simulink model "NInvState"  (R2024b)
settings: configuration reference "STM32H7_Config" (kept outside this file)
settings Model: DataDictionary=Master_Dictionary.sldd  EnableAccessToBaseWorkspace=off  Creator=torni  LastModifiedBy=William
settings ConfigSetRef: SourceName=STM32H7_Config

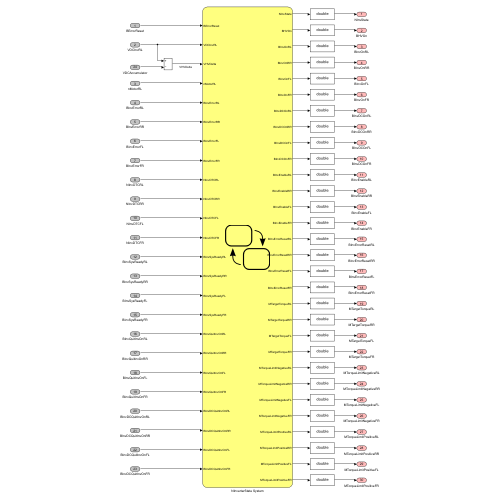
[thumbnail: Simulink's stored preview of the top-level diagram]
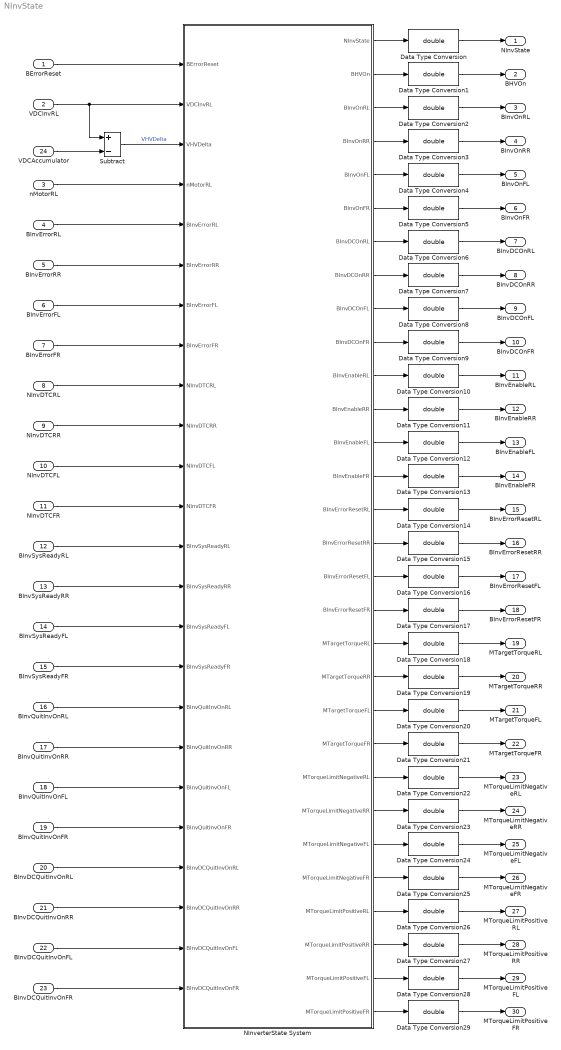
== system NInvState ==
  BErrorReset : Inport  OutDataTypeStr=boolean
  VDCInvRL : Inport  Port=2  OutDataTypeStr=double
  nMotorRL : Inport  Port=3  OutDataTypeStr=double
  BInvErrorRL : Inport  Port=4  OutDataTypeStr=boolean
  BInvErrorRR : Inport  Port=5  OutDataTypeStr=boolean
  BInvErrorFL : Inport  Port=6  OutDataTypeStr=boolean
  BInvErrorFR : Inport  Port=7  OutDataTypeStr=boolean
  NInvDTCRL : Inport  Port=8  OutDataTypeStr=double
  "NInvDTCRR " : Inport  Port=9  OutDataTypeStr=double
  NInvDTCFL : Inport  Port=10  OutDataTypeStr=double
  NInvDTCFR : Inport  Port=11  OutDataTypeStr=double
  BInvSysReadyRL : Inport  Port=12  OutDataTypeStr=boolean
  BInvSysReadyRR : Inport  Port=13  OutDataTypeStr=boolean
  BInvSysReadyFL : Inport  Port=14  OutDataTypeStr=boolean
  BInvSysReadyFR : Inport  Port=15  OutDataTypeStr=boolean
  BInvQuitInvOnRL : Inport  Port=16  OutDataTypeStr=boolean
  BInvQuitInvOnRR : Inport  Port=17  OutDataTypeStr=boolean
  BInvQuitInvOnFL : Inport  Port=18  OutDataTypeStr=boolean
  BInvQuitInvOnFR : Inport  Port=19  OutDataTypeStr=boolean
  BInvDCQuitInvOnRL : Inport  Port=20  OutDataTypeStr=boolean
  BInvDCQuitInvOnRR : Inport  Port=21  OutDataTypeStr=boolean
  BInvDCQuitInvOnFL : Inport  Port=22  OutDataTypeStr=boolean
  BInvDCQuitInvOnFR : Inport  Port=23  OutDataTypeStr=boolean
  VDCAccumulator : Inport  Port=24  OutDataTypeStr=double
  Data Type Conversion{,1..29} (30 alike) : DataTypeConversion  OutDataTypeStr=double  SaturateOnIntegerOverflow=off  RndMeth=Floor
  NInverterState System : Stateflow chart  TreatAsAtomicUnit=on
  Subtract : Sum  Inputs=+-
  NInvState : Outport  OutDataTypeStr=double  VectorParamsAs1DForOutWhenUnconnected=off
  BHVOn : Outport  Port=2  OutDataTypeStr=double  VectorParamsAs1DForOutWhenUnconnected=off
  BInvOnRL : Outport  Port=3  OutDataTypeStr=double  VectorParamsAs1DForOutWhenUnconnected=off
  BInvOnRR : Outport  Port=4  OutDataTypeStr=double  VectorParamsAs1DForOutWhenUnconnected=off
  BInvOnFL : Outport  Port=5  OutDataTypeStr=double  VectorParamsAs1DForOutWhenUnconnected=off
  BInvOnFR : Outport  Port=6  OutDataTypeStr=double  VectorParamsAs1DForOutWhenUnconnected=off
  BInvDCOnRL : Outport  Port=7  OutDataTypeStr=double  VectorParamsAs1DForOutWhenUnconnected=off
  BInvDCOnRR : Outport  Port=8  OutDataTypeStr=double  VectorParamsAs1DForOutWhenUnconnected=off
  BInvDCOnFL : Outport  Port=9  OutDataTypeStr=double  VectorParamsAs1DForOutWhenUnconnected=off
  BInvDCOnFR : Outport  Port=10  OutDataTypeStr=double  VectorParamsAs1DForOutWhenUnconnected=off
  BInvEnableRL : Outport  Port=11  OutDataTypeStr=double  VectorParamsAs1DForOutWhenUnconnected=off
  BInvEnableRR : Outport  Port=12  OutDataTypeStr=double  VectorParamsAs1DForOutWhenUnconnected=off
  BInvEnableFL : Outport  Port=13  OutDataTypeStr=double  VectorParamsAs1DForOutWhenUnconnected=off
  BInvEnableFR : Outport  Port=14  OutDataTypeStr=double  VectorParamsAs1DForOutWhenUnconnected=off
  BInvErrorResetRL : Outport  Port=15  OutDataTypeStr=double  VectorParamsAs1DForOutWhenUnconnected=off
  BInvErrorResetRR : Outport  Port=16  OutDataTypeStr=double  VectorParamsAs1DForOutWhenUnconnected=off
  BInvErrorResetFL : Outport  Port=17  OutDataTypeStr=double  VectorParamsAs1DForOutWhenUnconnected=off
  BInvErrorResetFR : Outport  Port=18  OutDataTypeStr=double  VectorParamsAs1DForOutWhenUnconnected=off
  MTargetTorqueRL : Outport  Port=19  OutDataTypeStr=double  VectorParamsAs1DForOutWhenUnconnected=off
  MTargetTorqueRR : Outport  Port=20  OutDataTypeStr=double  VectorParamsAs1DForOutWhenUnconnected=off
  MTargetTorqueFL : Outport  Port=21  OutDataTypeStr=double  VectorParamsAs1DForOutWhenUnconnected=off
  MTargetTorqueFR : Outport  Port=22  OutDataTypeStr=double  VectorParamsAs1DForOutWhenUnconnected=off
  MTorqueLimitNegativeRL : Outport  Port=23  OutDataTypeStr=double  VectorParamsAs1DForOutWhenUnconnected=off
  MTorqueLimitNegativeRR : Outport  Port=24  OutDataTypeStr=double  VectorParamsAs1DForOutWhenUnconnected=off
  MTorqueLimitNegativeFL : Outport  Port=25  OutDataTypeStr=double  VectorParamsAs1DForOutWhenUnconnected=off
  MTorqueLimitNegativeFR : Outport  Port=26  OutDataTypeStr=double  VectorParamsAs1DForOutWhenUnconnected=off
  MTorqueLimitPositiveRL : Outport  Port=27  OutDataTypeStr=double  VectorParamsAs1DForOutWhenUnconnected=off
  MTorqueLimitPositiveRR : Outport  Port=28  OutDataTypeStr=double  VectorParamsAs1DForOutWhenUnconnected=off
  MTorqueLimitPositiveFL : Outport  Port=29  OutDataTypeStr=double  VectorParamsAs1DForOutWhenUnconnected=off
  MTorqueLimitPositiveFR : Outport  Port=30  OutDataTypeStr=double  VectorParamsAs1DForOutWhenUnconnected=off
  wires:
  NInverterState System/2(BHVOn) -> Data Type Conversion1/1
  NInverterState System/1(NInvState) -> Data Type Conversion/1
  BErrorReset/1 -> NInverterState System/1(BErrorReset)
  VDCInvRL/1 -> NInverterState System/2(VDCInvRL), Subtract/1
  nMotorRL/1 -> NInverterState System/4(nMotorRL)
  BInvErrorRL/1 -> NInverterState System/5(BInvErrorRL)
  BInvErrorRR/1 -> NInverterState System/6(BInvErrorRR)
  BInvErrorFL/1 -> NInverterState System/7(BInvErrorFL)
  BInvErrorFR/1 -> NInverterState System/8(BInvErrorFR)
  NInvDTCRL/1 -> NInverterState System/9(NInvDTCRL)
  "NInvDTCRR "/1 -> NInverterState System/10(NInvDTCRR)
  NInvDTCFL/1 -> NInverterState System/11(NInvDTCFL)
  NInvDTCFR/1 -> NInverterState System/12(NInvDTCFR)
  BInvSysReadyRL/1 -> NInverterState System/13(BInvSysReadyRL)
  BInvSysReadyRR/1 -> NInverterState System/14(BInvSysReadyRR)
  BInvSysReadyFL/1 -> NInverterState System/15(BInvSysReadyFL)
  BInvSysReadyFR/1 -> NInverterState System/16(BInvSysReadyFR)
  BInvQuitInvOnRL/1 -> NInverterState System/17(BInvQuitInvOnRL)
  BInvQuitInvOnRR/1 -> NInverterState System/18(BInvQuitInvOnRR)
  BInvQuitInvOnFL/1 -> NInverterState System/19(BInvQuitInvOnFL)
  BInvQuitInvOnFR/1 -> NInverterState System/20(BInvQuitInvOnFR)
  BInvDCQuitInvOnRL/1 -> NInverterState System/21(BInvDCQuitInvOnRL)
  BInvDCQuitInvOnFL/1 -> NInverterState System/23(BInvDCQuitInvOnFL)
  BInvDCQuitInvOnRR/1 -> NInverterState System/22(BInvDCQuitInvOnRR)
  BInvDCQuitInvOnFR/1 -> NInverterState System/24(BInvDCQuitInvOnFR)
  VDCAccumulator/1 -> Subtract/2
  Subtract/1 -> NInverterState System/3(VHVDelta)  "VHVDelta"
  NInverterState System/19(MTargetTorqueRL) -> Data Type Conversion18/1
  NInverterState System/20(MTargetTorqueRR) -> Data Type Conversion19/1
  NInverterState System/21(MTargetTorqueFL) -> Data Type Conversion20/1
  NInverterState System/22(MTargetTorqueFR) -> Data Type Conversion21/1
  NInverterState System/23(MTorqueLimitNegativeRL) -> Data Type Conversion22/1
  NInverterState System/24(MTorqueLimitNegativeRR) -> Data Type Conversion23/1
  NInverterState System/25(MTorqueLimitNegativeFL) -> Data Type Conversion24/1
  NInverterState System/26(MTorqueLimitNegativeFR) -> Data Type Conversion25/1
  NInverterState System/27(MTorqueLimitPositiveRL) -> Data Type Conversion26/1
  NInverterState System/28(MTorqueLimitPositiveRR) -> Data Type Conversion27/1
  NInverterState System/29(MTorqueLimitPositiveFL) -> Data Type Conversion28/1
  NInverterState System/30(MTorqueLimitPositiveFR) -> Data Type Conversion29/1
  NInverterState System/18(BInvErrorResetFR) -> Data Type Conversion17/1
  NInverterState System/17(BInvErrorResetFL) -> Data Type Conversion16/1
  NInverterState System/16(BInvErrorResetRR) -> Data Type Conversion15/1
  NInverterState System/15(BInvErrorResetRL) -> Data Type Conversion14/1
  NInverterState System/14(BInvEnableFR) -> Data Type Conversion13/1
  NInverterState System/13(BInvEnableFL) -> Data Type Conversion12/1
  NInverterState System/12(BInvEnableRR) -> Data Type Conversion11/1
  NInverterState System/11(BInvEnableRL) -> Data Type Conversion10/1
  NInverterState System/10(BInvDCOnFR) -> Data Type Conversion9/1
  NInverterState System/9(BInvDCOnFL) -> Data Type Conversion8/1
  NInverterState System/8(BInvDCOnRR) -> Data Type Conversion7/1
  NInverterState System/7(BInvDCOnRL) -> Data Type Conversion6/1
  NInverterState System/6(BInvOnFR) -> Data Type Conversion5/1
  NInverterState System/5(BInvOnFL) -> Data Type Conversion4/1
  NInverterState System/4(BInvOnRR) -> Data Type Conversion3/1
  NInverterState System/3(BInvOnRL) -> Data Type Conversion2/1
  Data Type Conversion1/1 -> BHVOn/1
  Data Type Conversion/1 -> NInvState/1
  Data Type Conversion2/1 -> BInvOnRL/1
  Data Type Conversion3/1 -> BInvOnRR/1
  Data Type Conversion4/1 -> BInvOnFL/1
  Data Type Conversion5/1 -> BInvOnFR/1
  Data Type Conversion6/1 -> BInvDCOnRL/1
  Data Type Conversion7/1 -> BInvDCOnRR/1
  Data Type Conversion8/1 -> BInvDCOnFL/1
  Data Type Conversion9/1 -> BInvDCOnFR/1
  Data Type Conversion10/1 -> BInvEnableRL/1
  Data Type Conversion11/1 -> BInvEnableRR/1
  Data Type Conversion12/1 -> BInvEnableFL/1
  Data Type Conversion13/1 -> BInvEnableFR/1
  Data Type Conversion14/1 -> BInvErrorResetRL/1
  Data Type Conversion15/1 -> BInvErrorResetRR/1
  Data Type Conversion16/1 -> BInvErrorResetFL/1
  Data Type Conversion17/1 -> BInvErrorResetFR/1
  Data Type Conversion18/1 -> MTargetTorqueRL/1
  Data Type Conversion19/1 -> MTargetTorqueRR/1
  Data Type Conversion20/1 -> MTargetTorqueFL/1
  Data Type Conversion21/1 -> MTargetTorqueFR/1
  Data Type Conversion22/1 -> MTorqueLimitNegativeRL/1
  Data Type Conversion23/1 -> MTorqueLimitNegativeRR/1
  Data Type Conversion24/1 -> MTorqueLimitNegativeFL/1
  Data Type Conversion25/1 -> MTorqueLimitNegativeFR/1
  Data Type Conversion26/1 -> MTorqueLimitPositiveRL/1
  Data Type Conversion27/1 -> MTorqueLimitPositiveRR/1
  Data Type Conversion28/1 -> MTorqueLimitPositiveFL/1
  Data Type Conversion29/1 -> MTorqueLimitPositiveFR/1

== stateflow chart NInvState/NInverterState System ==
  state Inv_State_Idle
    entry:
    NInvState=0;
  state Inv_Error_Checks
    state Inv_LV_Check2
      entry:
      NInvState=2
      BInvErrorResetRR=0;
      BInvErrorResetRL=0;
      BInvErrorResetFR=0;
      BInvErrorResetFL=0;
    state Inv_LV_Check1
      entry:
      BInvErrorResetRR=1;
      BInvErrorResetRL=1;
      BInvErrorResetFR=1;
      BInvErrorResetFL=1;
    state Inv_LV_OK
      entry:
      NInvState=3;
    state Inv_LV_Check
      entry:
      NInvState=1;
      BInvErrorResetRR=0;
      BInvErrorResetRL=0;
      BInvErrorResetFR=0;
      BInvErrorResetFL=0;
    Inv_LV_Check1 -> Inv_LV_Check2 : after(100, tick)
        | [BInvErrorFL==0&&...
        | BInvErrorFR==0&&...
        | BInvErrorRR==0&&...
        | BInvErrorRL==0]
    (default) -> Inv_LV_Check
    Inv_LV_Check2 -> Inv_LV_Check [order 1] : [BInvErrorRR==1 &&...
        | BInvErrorRL==1 &&...
        | BInvErrorFR==1 &&...
        | BInvErrorFL==1]
    Inv_LV_Check2 -> Inv_LV_OK [order 2] : [BInvErrorRR==0 &&...
        | BInvErrorRL==0 &&...
        | BInvErrorFR==0 &&...
        | BInvErrorFL==0 &&...
        | BInvSysReadyRL==1 &&...
        | BInvSysReadyRR==1 &&...
        | BInvSysReadyFL==1 &&...
        | BInvSysReadyFR==1]
    Inv_LV_Check -> Inv_LV_Check1 : after(100,tick)
    Inv_LV_OK -> Inv_LV_Check : [BErrorReset==1 && nMotorRL<500]
  state Inv_OK
    entry:
    NInvState=92
  state Encoder_Reset_RL
    state Encoder_Error_RL
      entry:
      NInvState=404
      state PBX_SENSORS_ini
        entry:
        BInvErrorResetRL=0;
      state Error_On
        entry:
        BInvErrorResetRL=1;
      state Error_off
        entry:
        BInvErrorResetRL=0;
      (default) -> Encoder_Reset_RL.Encoder_Error_RL.PBX_SENSORS_ini
      Encoder_Reset_RL.Encoder_Error_RL.PBX_SENSORS_ini -> Encoder_Reset_RL.Encoder_Error_RL.Error_On : after(50, tick)
      Encoder_Reset_RL.Encoder_Error_RL.Error_off -> Encoder_Reset_RL.Encoder_Error_RL.PBX_SENSORS_ini [order 2] : [BInvErrorRL ==1]
      Encoder_Reset_RL.Encoder_Error_RL.Error_On -> Encoder_Reset_RL.Encoder_Error_RL.Error_off : after(100, tick)
          | [BInvErrorRL ==0]
    state Inverter_HV_Checks3
      exit:
      BHVOn=1
      state Inverter_IN
        entry:
        NInvState = 22
        BInvDCOnRL = 1
      state Inv_Error_Check_2
        BInvErrorResetRL = 0
        NInvState = 00
      state Inv_Error_Reset
        entry:
        NInvState = 00
        BInvErrorResetRL=1
        BInvDCOnRL=0
        BInvEnableRL = 0
        BInvOnRL = 0
      state START_UP
        entry:
        NInvState = 23
        MTargetTorqueRL=0
        MTorqueLimitNegativeRL = 0
        MTorqueLimitPositiveRL = 0
        BInvOnRL = 1
      state Inv_Error_Check_1
        entry:
        NInvState = 00
        MTorqueLimitNegativeRL = 0
        MTorqueLimitPositiveRL = 0
      state Inverter_ON
        entry:
        NInvState = 24
        BInvEnableRL = 1
      state TorqueReq_Ready
        entry:
        NInvState = 25
        MTorqueLimitNegativeRL = -100
        MTorqueLimitPositiveRL = 204.8
      (default) -> Encoder_Reset_RL.Inverter_HV_Checks3.Inverter_IN
      (junction 784) -> Encoder_Reset_RL.Inverter_HV_Checks3.Inverter_IN [order 1] : [BInvErrorRL==0]
      Encoder_Reset_RL.Inverter_HV_Checks3.Inv_Error_Check_2 -> (junction 784) : after(500,tick)
      (junction 784) -> Encoder_Reset_RL.Inverter_HV_Checks3.Inv_Error_Check_1 [order 2] : [BInvErrorRL==1]
      Encoder_Reset_RL.Inverter_HV_Checks3.Inv_Error_Reset -> Encoder_Reset_RL.Inverter_HV_Checks3.Inv_Error_Check_2 : after(500,tick)
      Encoder_Reset_RL.Inverter_HV_Checks3.Inverter_IN -> Encoder_Reset_RL.Inverter_HV_Checks3.START_UP : [BInvDCQuitInvOnRL==1]
      Encoder_Reset_RL.Inverter_HV_Checks3.START_UP -> Encoder_Reset_RL.Inverter_HV_Checks3.Inverter_ON : after(100,tick)
      Encoder_Reset_RL.Inverter_HV_Checks3.Inv_Error_Check_1 -> Encoder_Reset_RL.Inverter_HV_Checks3.Inv_Error_Reset : after(500,tick)
      Encoder_Reset_RL.Inverter_HV_Checks3.Inverter_ON -> Encoder_Reset_RL.Inverter_HV_Checks3.TorqueReq_Ready [order 1] : [BInvQuitInvOnRL == 1]
      Encoder_Reset_RL.Inverter_HV_Checks3.Inverter_ON -> Encoder_Reset_RL.Inverter_HV_Checks3.Inv_Error_Check_1 [order 2] : [BInvErrorRL==1]
      Encoder_Reset_RL.Inverter_HV_Checks3.TorqueReq_Ready -> Encoder_Reset_RL.Inverter_HV_Checks3.Inv_Error_Check_1 [order 1] : [BInvErrorRL==1]
    state Encoder_OK
      entry:
      NInvState = 26
    (default) -> Encoder_Error_RL
    Encoder_Reset_RL.Encoder_Error_RL.Error_off -> Encoder_Reset_RL.Inverter_HV_Checks3 [order 1] : [BInvSysReadyRL==1]
    Encoder_Reset_RL.Inverter_HV_Checks3.TorqueReq_Ready -> Encoder_Reset_RL.Encoder_OK [order 2] : [BInvErrorRL==0]
  state Encoder_Reset_RR
    state Encoder_Error_RR
      entry:
      NInvState = 404
      state PBX_SENSORS_ini
        entry:
        BInvErrorResetRR=0;
      state Error_On
        entry:
        BInvErrorResetRR=1;
      state Error_off
        entry:
        BInvErrorResetRR=0;
      (default) -> Encoder_Reset_RR.Encoder_Error_RR.PBX_SENSORS_ini
      Encoder_Reset_RR.Encoder_Error_RR.PBX_SENSORS_ini -> Encoder_Reset_RR.Encoder_Error_RR.Error_On : after(50, tick)
      Encoder_Reset_RR.Encoder_Error_RR.Error_off -> Encoder_Reset_RR.Encoder_Error_RR.PBX_SENSORS_ini [order 2] : [BInvErrorRR ==1]
      Encoder_Reset_RR.Encoder_Error_RR.Error_On -> Encoder_Reset_RR.Encoder_Error_RR.Error_off : after(100, tick)
          | [BInvErrorRR ==0]
    state Inverter_HV_CheckRR
      exit:
      BHVOn=1
      state Inverter_IN
        entry:
        NInvState = 27
        BInvDCOnRR = 1
      state Inv_Error_Check_2
        BInvErrorResetRR = 0
        NInvState = 00
      state Inv_Error_Reset
        entry:
        NInvState = 00
        BInvErrorResetRR=1
        BInvDCOnRR=0
        BInvEnableRR = 0
        BInvOnRR = 0
      state START_UP
        entry:
        NInvState = 28
        MTargetTorqueRR=0
        MTorqueLimitNegativeRR = 0
        MTorqueLimitPositiveRR = 0
        BInvOnRR = 1
      state Inv_Error_Check_1
        entry:
        NInvState = 00
        MTorqueLimitNegativeRR = 0
        MTorqueLimitPositiveRR = 0
      state Inverter_ON
        entry:
        NInvState = 29
        BInvEnableRR = 1
      state TorqueReq_Ready
        entry:
        NInvState = 30
        MTorqueLimitNegativeRR = -100
        MTorqueLimitPositiveRR = 204.8
      (default) -> Encoder_Reset_RR.Inverter_HV_CheckRR.Inverter_IN
      (junction 861) -> Encoder_Reset_RR.Inverter_HV_CheckRR.Inverter_IN [order 1] : [BInvErrorRR==0]
      Encoder_Reset_RR.Inverter_HV_CheckRR.Inv_Error_Check_2 -> (junction 861) : after(500,tick)
      (junction 861) -> Encoder_Reset_RR.Inverter_HV_CheckRR.Inv_Error_Check_1 [order 2] : [BInvErrorRR==1]
      Encoder_Reset_RR.Inverter_HV_CheckRR.Inv_Error_Reset -> Encoder_Reset_RR.Inverter_HV_CheckRR.Inv_Error_Check_2 : after(500,tick)
      Encoder_Reset_RR.Inverter_HV_CheckRR.Inverter_IN -> Encoder_Reset_RR.Inverter_HV_CheckRR.START_UP : [BInvDCQuitInvOnRR==1]
      Encoder_Reset_RR.Inverter_HV_CheckRR.START_UP -> Encoder_Reset_RR.Inverter_HV_CheckRR.Inverter_ON : after(100,tick)
      Encoder_Reset_RR.Inverter_HV_CheckRR.Inv_Error_Check_1 -> Encoder_Reset_RR.Inverter_HV_CheckRR.Inv_Error_Reset : after(500,tick)
      Encoder_Reset_RR.Inverter_HV_CheckRR.Inverter_ON -> Encoder_Reset_RR.Inverter_HV_CheckRR.TorqueReq_Ready [order 1] : [BInvQuitInvOnRR == 1]
      Encoder_Reset_RR.Inverter_HV_CheckRR.Inverter_ON -> Encoder_Reset_RR.Inverter_HV_CheckRR.Inv_Error_Check_1 [order 2] : [BInvErrorRR==1]
      Encoder_Reset_RR.Inverter_HV_CheckRR.TorqueReq_Ready -> Encoder_Reset_RR.Inverter_HV_CheckRR.Inv_Error_Check_1 [order 1] : [BInvErrorRR==1]
    state Encoder_OK
      entry:
      NInvState = 31
    (default) -> Encoder_Error_RR
    Encoder_Reset_RR.Encoder_Error_RR.Error_off -> Encoder_Reset_RR.Inverter_HV_CheckRR [order 1] : [BInvSysReadyRR==1]
    Encoder_Reset_RR.Inverter_HV_CheckRR.TorqueReq_Ready -> Encoder_Reset_RR.Encoder_OK [order 2] : [BInvErrorRR==0]
  state Encoder_Reset_FL
    state Encoder_Error_FL
      entry:
      NInvState = 404
      state Error_On
        entry:
        BInvErrorResetFL=1;
      state PBX_SENSORS_ini
        entry:
        BInvErrorResetFL=0;
      state Error_off
        entry:
        BInvErrorResetFL=0;
      (default) -> Encoder_Reset_FL.Encoder_Error_FL.PBX_SENSORS_ini
      Encoder_Reset_FL.Encoder_Error_FL.PBX_SENSORS_ini -> Encoder_Reset_FL.Encoder_Error_FL.Error_On : after(50, tick)
      Encoder_Reset_FL.Encoder_Error_FL.Error_off -> Encoder_Reset_FL.Encoder_Error_FL.PBX_SENSORS_ini [order 2] : [BInvErrorFL ==1]
      Encoder_Reset_FL.Encoder_Error_FL.Error_On -> Encoder_Reset_FL.Encoder_Error_FL.Error_off : after(100, tick)
          | [BInvErrorFL ==0]
    state Inverter_HV_Checks2
      exit:
      BHVOn=1
      state Inverter_IN
        entry:
        NInvState = 32
        BInvDCOnFL = 1
      state Inv_Error_Check_2
        BInvErrorResetFL = 0
        NInvState = 00
      state Inv_Error_Reset
        entry:
        NInvState = 00
        BInvErrorResetFL=1
        BInvDCOnFL=0
        BInvEnableFL = 0
        BInvOnFL = 0
      state START_UP
        entry:
        NInvState = 33
        MTargetTorqueFL=0
        MTorqueLimitNegativeFL = 0
        MTorqueLimitPositiveFL = 0
        BInvOnFL = 1
      state Inv_Error_Check_1
        entry:
        NInvState = 00
        MTorqueLimitNegativeFL = 0
        MTorqueLimitPositiveFL = 0
      state Inverter_ON
        entry:
        NInvState = 34
        BInvEnableFL = 1
      state TorqueReq_Ready
        entry:
        NInvState = 35
        MTorqueLimitNegativeFL = -100
        MTorqueLimitPositiveFL = 204.8
      (default) -> Encoder_Reset_FL.Inverter_HV_Checks2.Inverter_IN
      (junction 751) -> Encoder_Reset_FL.Inverter_HV_Checks2.Inverter_IN [order 1] : [BInvErrorFL==0]
      Encoder_Reset_FL.Inverter_HV_Checks2.Inv_Error_Check_2 -> (junction 751) : after(500,tick)
      (junction 751) -> Encoder_Reset_FL.Inverter_HV_Checks2.Inv_Error_Check_1 [order 2] : [BInvErrorFL==1]
      Encoder_Reset_FL.Inverter_HV_Checks2.Inv_Error_Reset -> Encoder_Reset_FL.Inverter_HV_Checks2.Inv_Error_Check_2 : after(500,tick)
      Encoder_Reset_FL.Inverter_HV_Checks2.Inverter_IN -> Encoder_Reset_FL.Inverter_HV_Checks2.START_UP : [BInvDCQuitInvOnFL==1]
      Encoder_Reset_FL.Inverter_HV_Checks2.START_UP -> Encoder_Reset_FL.Inverter_HV_Checks2.Inverter_ON : after(100,tick)
      Encoder_Reset_FL.Inverter_HV_Checks2.Inv_Error_Check_1 -> Encoder_Reset_FL.Inverter_HV_Checks2.Inv_Error_Reset : after(500,tick)
      Encoder_Reset_FL.Inverter_HV_Checks2.Inverter_ON -> Encoder_Reset_FL.Inverter_HV_Checks2.TorqueReq_Ready [order 1] : [BInvQuitInvOnFL == 1]
      Encoder_Reset_FL.Inverter_HV_Checks2.Inverter_ON -> Encoder_Reset_FL.Inverter_HV_Checks2.Inv_Error_Check_1 [order 2] : [BInvErrorFL==1]
      Encoder_Reset_FL.Inverter_HV_Checks2.TorqueReq_Ready -> Encoder_Reset_FL.Inverter_HV_Checks2.Inv_Error_Check_1 [order 1] : [BInvErrorFL==1]
    state Encoder_OK
      entry:
      NInvState = 36
    (default) -> Encoder_Error_FL
    Encoder_Reset_FL.Encoder_Error_FL.Error_off -> Inverter_HV_Checks2 [order 1] : [BInvSysReadyFL==1]
    Encoder_Reset_FL.Inverter_HV_Checks2.TorqueReq_Ready -> Encoder_Reset_FL.Encoder_OK [order 2] : [BInvErrorFL==0]
  state Inverter_HV_Checks
    state Inverter_HV_CheckFR
      exit:
      BHVOn=1;
      NInvState = 4
      state Inverter_IN
        entry:
        NInvState = 5
        BInvDCOnFR = 1
      state Inv_Error_Check_2
        BInvErrorResetFR = 0
        NInvState = 00;
      state Inv_Error_Reset
        entry:
        NInvState = 00
        BInvErrorResetFR=1
        BInvDCOnFR=0
        BInvEnableFR = 0
        BInvOnFR = 0
      state START_UP
        entry:
        NInvState = 6
        MTargetTorqueFR=0
        MTorqueLimitNegativeFR = 0
        MTorqueLimitPositiveFR = 0
        BInvOnFR = 1
      state Inv_Error_Check_1
        entry:
        NInvState = 00
        MTorqueLimitNegativeFR = 0
        MTorqueLimitPositiveFR = 0
      state Inverter_ON
        entry:
        NInvState = 7
        BInvEnableFR = 1
      state TorqueReq_Ready
        entry:
        NInvState = 8
        MTorqueLimitNegativeFR = -100
        MTorqueLimitPositiveFR = 204.8
      (default) -> Inverter_HV_Checks.Inverter_HV_CheckFR.Inverter_IN
      (junction 1179) -> Inverter_HV_Checks.Inverter_HV_CheckFR.Inverter_IN [order 1] : [BInvErrorFR==0]
      Inverter_HV_Checks.Inverter_HV_CheckFR.Inv_Error_Check_2 -> (junction 1179) : after(500,tick)
      (junction 1179) -> Inverter_HV_Checks.Inverter_HV_CheckFR.Inv_Error_Check_1 [order 2] : [BInvErrorFR==1]
      Inverter_HV_Checks.Inverter_HV_CheckFR.Inv_Error_Reset -> Inverter_HV_Checks.Inverter_HV_CheckFR.Inv_Error_Check_2 : after(500,tick)
      Inverter_HV_Checks.Inverter_HV_CheckFR.Inverter_IN -> Inverter_HV_Checks.Inverter_HV_CheckFR.START_UP : [BInvDCQuitInvOnFR==1]
      Inverter_HV_Checks.Inverter_HV_CheckFR.START_UP -> Inverter_HV_Checks.Inverter_HV_CheckFR.Inverter_ON : after(100,tick)
      Inverter_HV_Checks.Inverter_HV_CheckFR.Inv_Error_Check_1 -> Inverter_HV_Checks.Inverter_HV_CheckFR.Inv_Error_Reset : after(500,tick)
      Inverter_HV_Checks.Inverter_HV_CheckFR.Inverter_ON -> Inverter_HV_Checks.Inverter_HV_CheckFR.TorqueReq_Ready [order 1] : [BInvQuitInvOnFR == 1]
      Inverter_HV_Checks.Inverter_HV_CheckFR.Inverter_ON -> Inverter_HV_Checks.Inverter_HV_CheckFR.Inv_Error_Check_1 [order 2] : [BInvErrorFR==1]
      Inverter_HV_Checks.Inverter_HV_CheckFR.TorqueReq_Ready -> Inverter_HV_Checks.Inverter_HV_CheckFR.Inv_Error_Check_1 [order 2] : [BInvErrorFR==1]
    state Inv_HV_Check
    note: FRONT RIGHT INVERTER
    state Inverter_HV_CheckRR
      exit:
      BHVOn=1
      state Inverter_IN
        entry:
        NInvState = 9;
        BInvDCOnRR = 1
      state Inv_Error_Check_2
        BInvErrorResetRR = 0
      state Inv_Error_Reset
        entry:
        BInvErrorResetRR=1
        BInvDCOnRR=0
        BInvEnableRR = 0
        BInvOnRR = 0
      state START_UP
        entry:
        NInvState = 10
        MTargetTorqueRR=0
        MTorqueLimitNegativeRR = 0
        MTorqueLimitPositiveRR = 0
        BInvOnRR = 1
      state Inv_Error_Check_1
        entry:
        MTorqueLimitNegativeRR = 0
        MTorqueLimitPositiveRR = 0
      state Inverter_ON
        entry:
        NInvState = 11
        BInvEnableRR = 1
      state TorqueReq_Ready
        entry:
        NInvState = 12
        MTorqueLimitNegativeRR = -100
        MTorqueLimitPositiveRR = 204.8
      (default) -> Inverter_HV_Checks.Inverter_HV_CheckRR.Inverter_IN
      (junction 1201) -> Inverter_HV_Checks.Inverter_HV_CheckRR.Inverter_IN [order 1] : [BInvErrorRR==0]
      Inverter_HV_Checks.Inverter_HV_CheckRR.Inv_Error_Check_2 -> (junction 1201) : after(500,tick)
      (junction 1201) -> Inverter_HV_Checks.Inverter_HV_CheckRR.Inv_Error_Check_1 [order 2] : [BInvErrorRR==1]
      Inverter_HV_Checks.Inverter_HV_CheckRR.Inv_Error_Reset -> Inverter_HV_Checks.Inverter_HV_CheckRR.Inv_Error_Check_2 : after(500,tick)
      Inverter_HV_Checks.Inverter_HV_CheckRR.Inverter_IN -> Inverter_HV_Checks.Inverter_HV_CheckRR.START_UP : [BInvDCQuitInvOnRR==1]
      Inverter_HV_Checks.Inverter_HV_CheckRR.START_UP -> Inverter_HV_Checks.Inverter_HV_CheckRR.Inverter_ON : after(100,tick)
      Inverter_HV_Checks.Inverter_HV_CheckRR.Inv_Error_Check_1 -> Inverter_HV_Checks.Inverter_HV_CheckRR.Inv_Error_Reset : after(500,tick)
      Inverter_HV_Checks.Inverter_HV_CheckRR.Inverter_ON -> Inverter_HV_Checks.Inverter_HV_CheckRR.TorqueReq_Ready [order 1] : [BInvQuitInvOnRR == 1]
      Inverter_HV_Checks.Inverter_HV_CheckRR.Inverter_ON -> Inverter_HV_Checks.Inverter_HV_CheckRR.Inv_Error_Check_1 [order 2] : [BInvErrorRR==1]
      Inverter_HV_Checks.Inverter_HV_CheckRR.TorqueReq_Ready -> Inverter_HV_Checks.Inverter_HV_CheckRR.Inv_Error_Check_1 [order 2] : [BInvErrorRR==1]
    note: REAR RIGHT INVERTER
    state Inverter_HV_ChecksFL
      exit:
      BHVOn=1
      state Inverter_IN
        entry:
        NInvState = 13
        BInvDCOnFL = 1
      state Inv_Error_Check_2
        BInvErrorResetFL = 0
      state Inv_Error_Reset
        entry:
        BInvErrorResetFL=1
        BInvDCOnFL=0
        BInvEnableFL = 0
        BInvOnFL = 0
      state START_UP
        entry:
        NInvState = 14
        MTargetTorqueFL=0
        MTorqueLimitNegativeFL = 0
        MTorqueLimitPositiveFL = 0
        BInvOnFL = 1
      state Inv_Error_Check_1
        entry:
        MTorqueLimitNegativeFL = 0
        MTorqueLimitPositiveFL = 0
      state Inverter_ON
        entry:
        NInvState = 15
        BInvEnableFL = 1
      state TorqueReq_Ready
        entry:
        NInvState = 16
        MTorqueLimitNegativeFL = -100
        MTorqueLimitPositiveFL = 204.8
      (default) -> Inverter_HV_Checks.Inverter_HV_ChecksFL.Inverter_IN
      (junction 1222) -> Inverter_HV_Checks.Inverter_HV_ChecksFL.Inverter_IN [order 1] : [BInvErrorFL==0]
      Inverter_HV_Checks.Inverter_HV_ChecksFL.Inv_Error_Check_2 -> (junction 1222) : after(500,tick)
      (junction 1222) -> Inverter_HV_Checks.Inverter_HV_ChecksFL.Inv_Error_Check_1 [order 2] : [BInvErrorFL==1]
      Inverter_HV_Checks.Inverter_HV_ChecksFL.Inv_Error_Reset -> Inverter_HV_Checks.Inverter_HV_ChecksFL.Inv_Error_Check_2 : after(500,tick)
      Inverter_HV_Checks.Inverter_HV_ChecksFL.Inverter_IN -> Inverter_HV_Checks.Inverter_HV_ChecksFL.START_UP : [BInvDCQuitInvOnFL==1]
      Inverter_HV_Checks.Inverter_HV_ChecksFL.START_UP -> Inverter_HV_Checks.Inverter_HV_ChecksFL.Inverter_ON : after(100,tick)
      Inverter_HV_Checks.Inverter_HV_ChecksFL.Inv_Error_Check_1 -> Inverter_HV_Checks.Inverter_HV_ChecksFL.Inv_Error_Reset : after(500,tick)
      Inverter_HV_Checks.Inverter_HV_ChecksFL.Inverter_ON -> Inverter_HV_Checks.Inverter_HV_ChecksFL.TorqueReq_Ready [order 1] : [BInvQuitInvOnFL == 1]
      Inverter_HV_Checks.Inverter_HV_ChecksFL.Inverter_ON -> Inverter_HV_Checks.Inverter_HV_ChecksFL.Inv_Error_Check_1 [order 2] : [BInvErrorFL==1]
      Inverter_HV_Checks.Inverter_HV_ChecksFL.TorqueReq_Ready -> Inverter_HV_Checks.Inverter_HV_ChecksFL.Inv_Error_Check_1 [order 2] : [BInvErrorFL==1]
    note: FRONT LEFT INVERTER
    state Inverter_HV_ChecksRL
      exit:
      BHVOn=1
      state Inverter_IN
        entry:
        NInvState = 17
        BInvDCOnRL = 1
      state Inv_Error_Check_2
        BInvErrorResetRL = 0
      state Inv_Error_Reset
        entry:
        BInvErrorResetRL=1
        BInvDCOnRL=0
        BInvEnableRL = 0
        BInvOnRL = 0
      state START_UP
        entry:
        NInvState = 18
        MTargetTorqueRL=0
        MTorqueLimitNegativeRL = 0
        MTorqueLimitPositiveRL = 0
        BInvOnRL = 1
      state Inv_Error_Check_1
        entry:
        MTorqueLimitNegativeRL = 0
        MTorqueLimitPositiveRL = 0
      state Inverter_ON
        entry:
        NInvState = 19
        BInvEnableRL = 1
      state TorqueReq_Ready
        entry:
        NInvState = 20
        MTorqueLimitNegativeRL = -100
        MTorqueLimitPositiveRL = 204.8
      (default) -> Inverter_HV_Checks.Inverter_HV_ChecksRL.Inverter_IN
      (junction 1243) -> Inverter_HV_Checks.Inverter_HV_ChecksRL.Inverter_IN [order 1] : [BInvErrorRL==0]
      Inverter_HV_Checks.Inverter_HV_ChecksRL.Inv_Error_Check_2 -> (junction 1243) : after(500,tick)
      (junction 1243) -> Inverter_HV_Checks.Inverter_HV_ChecksRL.Inv_Error_Check_1 [order 2] : [BInvErrorRL==1]
      Inverter_HV_Checks.Inverter_HV_ChecksRL.Inv_Error_Reset -> Inverter_HV_Checks.Inverter_HV_ChecksRL.Inv_Error_Check_2 : after(500,tick)
      Inverter_HV_Checks.Inverter_HV_ChecksRL.Inverter_IN -> Inverter_HV_Checks.Inverter_HV_ChecksRL.START_UP : [BInvDCQuitInvOnRL==1]
      Inverter_HV_Checks.Inverter_HV_ChecksRL.START_UP -> Inverter_HV_Checks.Inverter_HV_ChecksRL.Inverter_ON : after(100,tick)
      Inverter_HV_Checks.Inverter_HV_ChecksRL.Inv_Error_Check_1 -> Inverter_HV_Checks.Inverter_HV_ChecksRL.Inv_Error_Reset : after(500,tick)
      Inverter_HV_Checks.Inverter_HV_ChecksRL.Inverter_ON -> Inverter_HV_Checks.Inverter_HV_ChecksRL.TorqueReq_Ready [order 1] : [BInvQuitInvOnRL == 1]
      Inverter_HV_Checks.Inverter_HV_ChecksRL.Inverter_ON -> Inverter_HV_Checks.Inverter_HV_ChecksRL.Inv_Error_Check_1 [order 2] : [BInvErrorRL==1]
      Inverter_HV_Checks.Inverter_HV_ChecksRL.TorqueReq_Ready -> Inverter_HV_Checks.Inverter_HV_ChecksRL.Inv_Error_Check_1 [order 1] : [BInvErrorRL==1]
    note: REAR LEFT INVERTER
    state Inv_OK
      entry:
      NInvState = 21;
    (default) -> Inv_HV_Check
    Inv_HV_Check -> Inverter_HV_CheckFR : [NInvState==3]
    Inverter_HV_Checks.Inverter_HV_CheckFR.TorqueReq_Ready -> Inverter_HV_Checks.Inverter_HV_CheckRR [order 1] : after(500,tick)[BInvErrorFR==0]
    Inverter_HV_Checks.Inverter_HV_CheckRR.TorqueReq_Ready -> Inverter_HV_ChecksFL [order 1] : after(500,tick)[BInvErrorRR==0]
    Inverter_HV_Checks.Inverter_HV_ChecksFL.TorqueReq_Ready -> Inverter_HV_ChecksRL [order 1] : after(500,tick)[BInvErrorFL==0]
    Inverter_HV_Checks.Inverter_HV_ChecksRL.TorqueReq_Ready -> Inverter_HV_Checks.Inv_OK [order 2] : [BInvErrorRL==0]
  state Encoder_Reset_FR
    state Encoder_Error_FR
      entry:
      NInvState = 404
      state PBX_SENSORS_ini
        entry:
        BInvErrorResetFR=0;
      state Error_On
        entry:
        BInvErrorResetFR=1;
      state Error_off
        entry:
        BInvErrorResetFR=0;
      (default) -> Encoder_Reset_FR.Encoder_Error_FR.PBX_SENSORS_ini
      Encoder_Reset_FR.Encoder_Error_FR.PBX_SENSORS_ini -> Encoder_Reset_FR.Encoder_Error_FR.Error_On : after(50, tick)
      Encoder_Reset_FR.Encoder_Error_FR.Error_off -> Encoder_Reset_FR.Encoder_Error_FR.PBX_SENSORS_ini [order 2] : [BInvErrorFR ==1]
      Encoder_Reset_FR.Encoder_Error_FR.Error_On -> Encoder_Reset_FR.Encoder_Error_FR.Error_off : after(100, tick)
          | [BInvErrorFR ==0]
    state Inverter_HV_Checks3
      exit:
      BHVOn=1
      state Inverter_IN
        entry:
        NInvState = 37
        BInvDCOnFR = 1
      state Inv_Error_Check_2
        BInvErrorResetFR = 0
        NInvState = 00
      state Inv_Error_Reset
        entry:
        NInvState = 00
        BInvErrorResetFR=1
        BInvDCOnFR=0
        BInvEnableFR = 0
        BInvOnFR = 0
      state START_UP
        entry:
        NInvState = 38
        MTargetTorqueFR=0
        MTorqueLimitNegativeFR = 0
        MTorqueLimitPositiveFR = 0
        BInvOnFR = 1
      state Inv_Error_Check_1
        entry:
        NInvState = 00
        MTorqueLimitNegativeFR = 0
        MTorqueLimitPositiveFR = 0
      state Inverter_ON
        entry:
        NInvState = 39
        BInvEnableFR = 1
      state TorqueReq_Ready
        entry:
        NInvState = 40
        MTorqueLimitNegativeFR = -100
        MTorqueLimitPositiveFR = 204.8
      (default) -> Encoder_Reset_FR.Inverter_HV_Checks3.Inverter_IN
      (junction 718) -> Encoder_Reset_FR.Inverter_HV_Checks3.Inverter_IN [order 1] : [BInvErrorFR==0]
      Encoder_Reset_FR.Inverter_HV_Checks3.Inv_Error_Check_2 -> (junction 718) : after(500,tick)
      (junction 718) -> Encoder_Reset_FR.Inverter_HV_Checks3.Inv_Error_Check_1 [order 2] : [BInvErrorFR==1]
      Encoder_Reset_FR.Inverter_HV_Checks3.Inv_Error_Reset -> Encoder_Reset_FR.Inverter_HV_Checks3.Inv_Error_Check_2 : after(500,tick)
      Encoder_Reset_FR.Inverter_HV_Checks3.Inverter_IN -> Encoder_Reset_FR.Inverter_HV_Checks3.START_UP : [BInvDCQuitInvOnFR==1]
      Encoder_Reset_FR.Inverter_HV_Checks3.START_UP -> Encoder_Reset_FR.Inverter_HV_Checks3.Inverter_ON : after(100,tick)
      Encoder_Reset_FR.Inverter_HV_Checks3.Inv_Error_Check_1 -> Encoder_Reset_FR.Inverter_HV_Checks3.Inv_Error_Reset : after(500,tick)
      Encoder_Reset_FR.Inverter_HV_Checks3.Inverter_ON -> Encoder_Reset_FR.Inverter_HV_Checks3.TorqueReq_Ready [order 1] : [BInvQuitInvOnFR == 1]
      Encoder_Reset_FR.Inverter_HV_Checks3.Inverter_ON -> Encoder_Reset_FR.Inverter_HV_Checks3.Inv_Error_Check_1 [order 2] : [BInvErrorFR==1]
      Encoder_Reset_FR.Inverter_HV_Checks3.TorqueReq_Ready -> Encoder_Reset_FR.Inverter_HV_Checks3.Inv_Error_Check_1 [order 1] : [BInvErrorFR==1]
    state Encoder_OK
      entry:
      NInvState = 41
    (default) -> Encoder_Error_FR
    Encoder_Reset_FR.Encoder_Error_FR.Error_off -> Encoder_Reset_FR.Inverter_HV_Checks3 [order 1] : [BInvSysReadyFR==1]
    Encoder_Reset_FR.Inverter_HV_Checks3.TorqueReq_Ready -> Encoder_Reset_FR.Encoder_OK [order 2] : [BInvErrorFR==0]
  (default) -> Inv_State_Idle
  Inv_State_Idle -> Inv_Error_Checks : [after (7000,tick)]
  Inv_OK -> Inv_State_Idle [order 6] : [VDCInvRL<60]
  Inv_OK -> Inv_Error_Checks [order 1] : [BErrorReset==1]
  Encoder_Reset_RL -> Inv_OK : [NInvState == 26]
  Inv_OK -> Encoder_Reset_RL [order 3] : [NInvDTCRL~=0 &&...
      | NInvDTCRL~=1049]
  Inverter_HV_Checks -> Inv_Error_Checks [order 1] : [BErrorReset==1]
  Inv_Error_Checks -> Inverter_HV_Checks : [VDCInvRL>60&&...
      | abs(VHVDelta)<10]
  Encoder_Reset_RR -> Inv_OK : [NInvState == 31]
  Inv_OK -> Encoder_Reset_RR [order 5] : [NInvDTCRR~=0 &&...
      | NInvDTCRR~=1049]
  Encoder_Reset_FL -> Inv_OK : [NInvState == 36]
  Inv_OK -> Encoder_Reset_FL [order 4] : [NInvDTCFL~=0 &&...
      | NInvDTCFL~=1049]
  Inverter_HV_Checks -> Inv_OK [order 2] : [NInvState==21]
  Encoder_Reset_FR -> Inv_OK : [NInvState == 41]
  Inv_OK -> Encoder_Reset_FR [order 2] : [NInvDTCFR~=0 &&...
      | NInvDTCFR~=1049]
  data: NInvState output double; BErrorReset input boolean; VDCInvRL input double; VHVDelta input double; nMotorRL input double; BInvErrorRL input boolean; BInvErrorRR input boolean; BInvErrorFL input boolean; BInvErrorFR input boolean; NInvDTCRL input double; NInvDTCRR input double; NInvDTCFL input double; NInvDTCFR input double; BInvSysReadyRL input boolean; BInvSysReadyRR input boolean; BInvSysReadyFL input boolean; BInvSysReadyFR input boolean; BInvQuitInvOnRL input boolean; BInvQuitInvOnRR input boolean; BInvQuitInvOnFL input boolean; BInvQuitInvOnFR input boolean; BInvDCQuitInvOnRL input boolean; BInvDCQuitInvOnRR input boolean; BHVOn output double; BInvOnRL output double; BInvOnRR output double; BInvOnFL output double; BInvOnFR output double; BInvDCOnRL output double; BInvDCOnRR output double; BInvDCOnFL output double; BInvDCOnFR output double; BInvEnableRL output double; BInvEnableRR output double; BInvEnableFL output double; BInvEnableFR output double; BInvErrorResetRL output double; BInvErrorResetRR output double; BInvErrorResetFL output double; BInvErrorResetFR output double; MTargetTorqueRL output double; MTargetTorqueRR output double; MTargetTorqueFL output double; MTargetTorqueFR output double; MTorqueLimitNegativeRL output double; MTorqueLimitNegativeRR output double; BInvDCQuitInvOnFL input boolean; MTorqueLimitNegativeFL output double; MTorqueLimitNegativeFR output double; MTorqueLimitPositiveRL output double; MTorqueLimitPositiveRR output double; MTorqueLimitPositiveFL output double; BInvDCQuitInvOnFR input boolean; MTorqueLimitPositiveFR output double
